simulink model "Model"  (R2024b)
settings: Solver=ode45  StartTime=0.0  StopTime=10  MaxStep=0.001  RelTol=1e-3
InitFcn:
  | Design
values from neighbouring files (symbols this model uses):
  Kw = 1 / Tw    (= 7.14285714286)    [Design.m]
  Mp = 0.3    [Design.m]
  P = (1 / (N * s)) * (kdrv * Kt * (Jb * s^2 + Bb * s + k))      / ((Req * D_tau_prime)      + Kt * Ke * (Jb * s^2 + Bb * s + k))    [Design.m]
  Ref = 50    [Design.m]
undefined symbols (not defined in the file or in its folder): daq, drv, ElecDyn, gbox, InternalTs, Kd, Ki, Kp, MechDyn, mld, mot, rads2rpm, sens, Tau_sf, Tl
libraries: simulink_extras x5
settings Model: Creator=Banaan  LastModifiedBy=Banaan

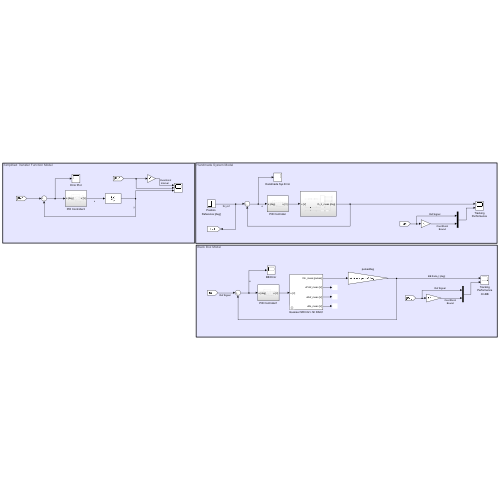
[thumbnail: Simulink's stored preview of the top-level diagram]
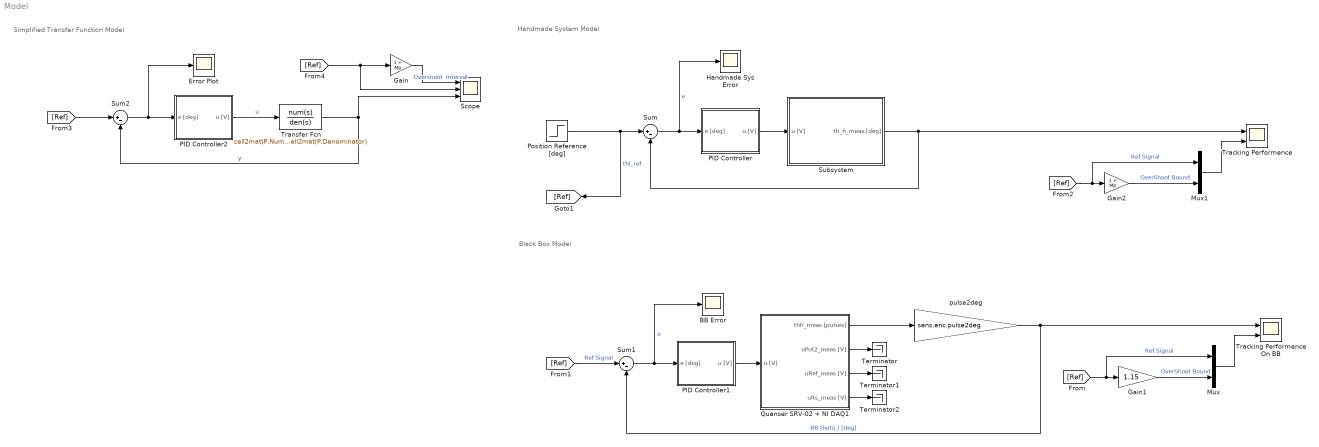
== system Model ==
  note: Simplified Transfer Function Model
  note: Handmade System Model
  note: Black Box Model
  BB Error : Scope
  Error Plot : Scope
  Gain : Gain  Gain=1 + Mp
  Gain1 : Gain  Gain=1.15
  Gain2 : Gain  Gain=1 + Mp
  Handmade Sys Error : Scope
  Mux : Mux  Inputs=2
  Mux1 : Mux  Inputs=2
  PID Controller : Subsystem
  PID Controller1 : Subsystem
  PID Controller2 : Subsystem
  Position Reference [deg] : Step  After=Ref  SampleTime=0
  Quanser SRV-02 + NI DAQ1 : Subsystem  mask(Quanser SRV-02 (with resonant load) + NI DAQ){Ts=0.001, fricType=Coulomb + viscous, lockShaft=off, beamInitPos=10}
      mask prompts: Ts "NI DAQ Sample Time:"; fricType "Friction model"; lockShaft "Lock motor shaft"; beamInitPos "Beam initial position [deg]:"
      mask help: Quanser SRV-02 (with resonant load) + NI DAQ model.
      mask init:
      | %%
      | % Riccardo Antonello (riccardo.antonello@unipd.it)
      | %
      | % April 28, 2020
      | %
      | % Dept. of Information Engineering, University of Padova
      | %
      | 
      | %%  Conversion gains
      | deg2rad = pi/180;                   %   [deg]   -> [rad]
      | rad2deg = 180/pi;                   %   [rad]   -> [deg]
      | 
      | 
      | %%  Sensors data
      | 
      | %   shunt resistor
      | sens.curr.Rs = 0.5;   
      | 
      | %   Hewlett-Packard HEDS-5540#A06 optical encoder
      | sens.enc.ppr = 500*4;                                                   %   pulses per rotation
      | sens.enc.pulse2deg = 360/sens.enc.ppr;                                  %   [pulses] -> [deg]
      | sens.enc.pulse2rad = 2*pi/sens.enc.ppr;                                 %   [pulses] -> [rad]
      | sens.enc.deg2pulse = sens.enc.ppr/360;                                  %   [deg] -> [pulses]
      | sens.enc.rad2pulse = sens.enc.ppr/2/pi;                                 %   [rad] -> [pulses]
      | 
      | %   potentiometer 2 (Spectrol 357-0-0-103) - installed on hub
      | sens.pot2.range.R      = 10e3;                                          %   ohmic value range 
      | sens.pot2.range.V      = 5;                                             %   voltage range
      | sens.pot2.range.th_deg = 340;                                           %   angle range [deg]
      | sens.pot2.range.th     = sens.pot2.range.th_deg * deg2rad;              %   angle range [rad]                           
      | sens.pot2.deg2V        = sens.pot2.range.V / sens.pot2.range.th_deg;    %   sensitivity [V/deg]
      | sens.pot2.rad2V        = sens.pot2.range.V / sens.pot2.range.th;        %   sensitivity [V/rad]
      | sens.pot2.V2deg        = 1/sens.pot2.deg2V;                             %   conversion gain [V] -> [deg]
      | sens.pot2.V2rad        = 1/sens.pot2.rad2V;                             %   conversion gain [V] -> [rad]
      | sens.pot2.noise.var    = 3.5e-7;                                        %   out noise variance [V^2]
      | 
      | 
      | %%  Data acquisition board (daq) data
      | 
      | %   NI PCI-6221 DAC data
      | daq.dac.bits = 16;                                  %   resolution (bits)
      | daq.dac.fs   = 10;                                  %   full scale 
      | daq.dac.q    = 2*daq.dac.fs/(2^daq.dac.bits-1);     %	quantization
      | 
      | %   NI PCI-6221 ADC data
      | daq.adc.bits = 16;                                  %   resolution (bits)
      | daq.adc.fs   = 10;                                  %   full scale (as set in SLDRT Analog Input block)
      | daq.adc.q    = 2*daq.adc.fs/(2^daq.adc.bits-1);     %   quantization   
      | 
      | 
      | %%  Set beam initial position
      | % SRV02Handle = find_system(gcb, ...
      | %     'LookUnderMasks', 'on', ...
      | %     'FindAll', 'on', ...
      | %     'FollowLinks', 'on', ...
      | %     'SearchDepth', '1', ...
      | %     'BlockType', 'ModelReference', ...
      | %     'Name', 'Quanser SRV-02');
      | %
      | % %get_param(SRV02Handle, 'InstanceParameters')
      | % InstanceParams = get_param(SRV02Handle, 'InstanceParameters');
      | % for k = 1:length(InstanceParams)
      | %     if strcmp(InstanceParams(k).Name, 'thb0')
      | %         if lockShaft
      | %             InstanceParams(k).Value = sprintf('%f', beamInitPos);
      | %         else
      | %             InstanceParams(k).Value = sprintf('%f', 0);    
      | %         end
      | %         set_param(SRV02Handle, 'InstanceParameters', InstanceParams);
      | %         break;
      | %     end
      | % end
      | 
      | if lockShaft
      |     thb0 = beamInitPos;
      | else
      |     thb0 = 0;    
      | end
      | 
      | 
      | %%  Mask initialization
      | if lockShaft
      |     
      |     %   find Inport handle
      |     InPortHandle = find_system(gcb, ...
      |         'LookUnderMasks', 'on', ...
      |         'FindAll', 'on', ...
      |         'FollowLinks', 'on', ...
      |         'SearchDepth', '1', ...
      |         'BlockType', 'Inport', ...
      |         'Name', 'u [V]');
      |     
      |     if ~isempty(InPortHandle)
      |     
      |         %   find DAC handle
      |         DACHandle = find_system(gcb, ...
      |             'LookUnderMasks', 'on', ...
      |             'FindAll', 'on', ...
      |             'FollowLinks', 'on', ...
      |             'SearchDepth', '1', ...
      |             'BlockType', 'SubSystem', ...
      |             'Name', 'DAC');  
      | 
      |         %   remove Inport output connection   
      |         InportConn = get_param(InPortHandle, 'PortConnectivity');
      |         delete_line(gcb, InportConn.Position);
      | 
      |         %   remove Inport block
      |         delete_block(InPortHandle);
      | 
      |         %   add Constant block
      |         ConstantHandle = add_block( ...
      |             'simulink/Sources/Constant', [gcb, '/u [V]'], ...
      |             'Position', [20   -37    50   -23], ...
      |             'Value', '0');
      | 
      |         %   connect Constant to DAC block
      |         DACPortHandles = get_param(DACHandle, 'PortHandles');
      |         ConstantPortHandles = get_param(ConstantHandle, 'PortHandles');
      |         add_line(gcb, ConstantPortHandles.Outport(1), DACPortHandles.Inport(1));
      |     
      |     end
      |     
      | else
      |     
      |     %   find Constant handle
      |     ConstantHandle = find_system(gcb, ...
      |         'LookUnderMasks', 'on', ...
      |         'FindAll', 'on', ...
      |         'FollowLinks', 'on', ...
      |         'SearchDepth', '1', ...
      |         'BlockType', 'Constant', ...
      |         'Name', 'u [V]');
      |     
      |     if ~isempty(ConstantHandle)
      |     
      |         %   find DAC handle
      |         DACHandle = find_system(gcb, ...
      |             'LookUnderMasks', 'on', ...
      |             'FindAll', 'on', ...
      |             'FollowLinks', 'on', ...
      |             'SearchDepth', '1', ...
      |             'BlockType', 'SubSystem', ...
      |             'Name', 'DAC');  
      |  
      |         %   remove Constant output connection   
      |         ConstantConn = get_param(ConstantHandle, 'PortConnectivity');
      |         delete_line(gcb, ConstantConn.Position);
      | 
      |         %   remove Inport block
      |         delete_block(ConstantHandle);   
      | 
      |         %   add Inport block
      |         InportHandle = add_block( ...
      |             'simulink/Sources/In1', [gcb, '/u [V]'], ...
      |             'Position', [20   -37    50   -23], ...
      |             'Port', '1');
      | 
      |         %   connect Constant to DAC block
      |         DACPortHandles = get_param(DACHandle, 'PortHandles');
      |         InportPortHandles = get_param(InportHandle, 'PortHandles');
      |         add_line(gcb, InportPortHandles.Outport(1), DACPortHandles.Inport(1));
      |     
      |      end
      |     
      | end
      mask Help:
      | Riccardo Antonello (antonello@dei.unipd.it)
      | 
      | April 28, 2020
      | 
      | Dept. of Information Engineering, University of Padova
      mask TypeOptions fricType: Coulomb + viscous | Karnopp
      mask Callback lockShaft:
      | %   get status of check box
      | lockShaft = get_param(gcb, 'lockShaft');
      | 
      | %   get current value of MaskVisibilities property
      | maskVisibilities = get_param(gcb, 'MaskVisibilities');
      | 
      | %   set visibility of the dialog box element
      | if strcmp(lockShaft, 'on')
      |     maskVisibilities{4} = 'on';
      | else
      |     maskVisibilities{4} = 'off';
      | end
      | 
      | % Set the 'MaskVisibilities' property for each parameter in mask
      | set_param( gcb, 'MaskVisibilities', maskVisibilities);
  Scope : Scope  NumInputPorts=3
  Subsystem : Subsystem
  Sum : Sum  Inputs=|+-
  Sum1 : Sum  Inputs=|+-
  Sum2 : Sum  Inputs=|+-
  Terminator : Terminator
  Terminator1 : Terminator
  Terminator2 : Terminator
  Tracking Performence : Scope  NumInputPorts=2
  Tracking Performence On BB : Scope  NumInputPorts=2
  Transfer Fcn : TransferFcn  Numerator=cell2mat(P.Numerator)  Denominator=cell2mat(P.Denominator)
  pulse2deg : Gain  Gain=sens.enc.pulse2deg
  wires:
  PID Controller/1(u [V]) -> Subsystem/1(u [V])
  Sum/1 -> PID Controller/1(e [deg]), Handmade Sys Error/1  "e"
  Subsystem/1(th_h_meas [deg]) -> Tracking Performence/1, Sum/2
  Position Reference [deg]/1 -> [Ref], Sum/1  "thl_ref"
  Quanser SRV-02 + NI DAQ1/1(thh_meas [pulses]) -> pulse2deg/1
  pulse2deg/1 -> Tracking Performence On BB/1, Sum1/2  "BB theta_l [deg]"
  Sum1/1 -> PID Controller1/1(e [deg]), BB Error/1  "e"
  PID Controller1/1(u [V]) -> Quanser SRV-02 + NI DAQ1/1(u [V])
  Gain1/1 -> Mux/2  "OverShoot Bound"
  [Ref] -> Mux/1, Gain1/1  "Ref Signal"
  Mux/1 -> Tracking Performence On BB/2
  [Ref] -> Sum1/1  "Ref Signal"
  Mux1/1 -> Tracking Performence/2
  [Ref] -> Gain2/1, Mux1/1  "Ref Signal"
  Gain2/1 -> Mux1/2  "OverShoot Bound"
  PID Controller2/1(u [V]) -> Transfer Fcn/1  "u"
  [Ref] -> Sum2/1
  Sum2/1 -> Error Plot/1, PID Controller2/1(e [deg])
  Transfer Fcn/1 -> Sum2/2, Scope/3  "y"
  Gain/1 -> Scope/1  "Overshoot  Interval"
  [Ref] -> Scope/2, Gain/1
  Quanser SRV-02 + NI DAQ1/3(uRef_meas [V]) -> Terminator1/1
  Quanser SRV-02 + NI DAQ1/2(uPot2_meas [V]) -> Terminator/1
  Quanser SRV-02 + NI DAQ1/4(uRs_meas [V]) -> Terminator2/1

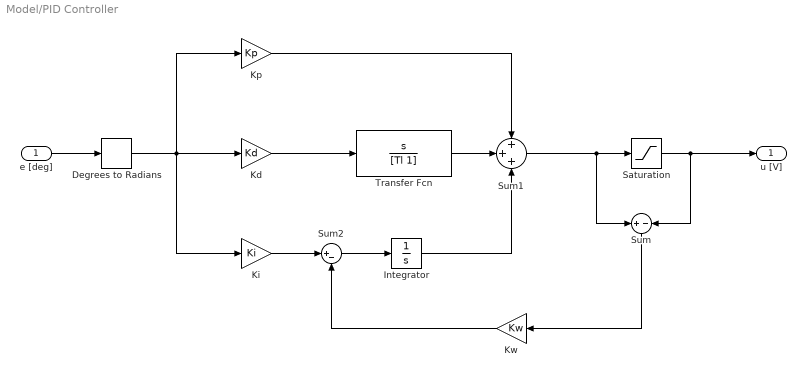
== system Model/PID Controller ==
  e [deg] : Inport
  Degrees to Radians : simulink_extras/Transformations/Degrees to Radians
  Integrator : Integrator
  Kd : Gain  Gain=Kd
  Ki : Gain  Gain=Ki
  Kp : Gain  Gain=Kp
  Kw : Gain  Gain=Kw
  Saturation : Saturate  UpperLimit=daq.dac.fs  LowerLimit=-daq.dac.fs
  Sum : Sum  Inputs=+|-
  Sum1 : Sum  Inputs=+++
  Sum2 : Sum  Inputs=|+-
  Transfer Fcn : TransferFcn  Numerator=[1 0]  Denominator=[Tl 1]
  u [V] : Outport
  wires:
  Integrator/1 -> Sum1/3
  Sum2/1 -> Integrator/1
  Sum1/1 -> Sum/1, Saturation/1
  Ki/1 -> Sum2/1
  Kw/1 -> Sum2/2
  Kp/1 -> Sum1/1
  Sum/1 -> Kw/1
  Transfer Fcn/1 -> Sum1/2
  e [deg]/1 -> Degrees to Radians/1
  Kd/1 -> Transfer Fcn/1
  Saturation/1 -> u [V]/1, Sum/2
  Degrees to Radians/1 -> Kp/1, Kd/1, Ki/1

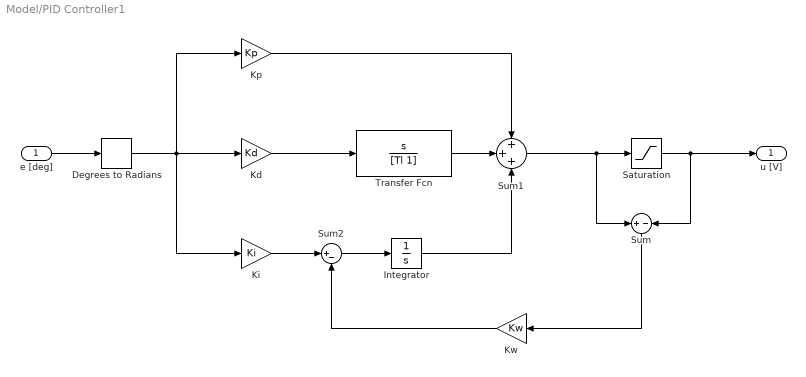
== system Model/PID Controller1 ==
  e [deg] : Inport
  Degrees to Radians : simulink_extras/Transformations/Degrees to Radians
  Integrator : Integrator
  Kd : Gain  Gain=Kd
  Ki : Gain  Gain=Ki
  Kp : Gain  Gain=Kp
  Kw : Gain  Gain=Kw
  Saturation : Saturate  UpperLimit=daq.dac.fs  LowerLimit=-daq.dac.fs
  Sum : Sum  Inputs=+|-
  Sum1 : Sum  Inputs=+++
  Sum2 : Sum  Inputs=|+-
  Transfer Fcn : TransferFcn  Numerator=[1 0]  Denominator=[Tl 1]
  u [V] : Outport
  wires:
  Kp/1 -> Sum1/1
  Degrees to Radians/1 -> Kp/1, Kd/1, Ki/1
  e [deg]/1 -> Degrees to Radians/1
  Saturation/1 -> u [V]/1, Sum/2
  Transfer Fcn/1 -> Sum1/2
  Sum2/1 -> Integrator/1
  Kd/1 -> Transfer Fcn/1
  Sum1/1 -> Sum/1, Saturation/1
  Sum/1 -> Kw/1
  Integrator/1 -> Sum1/3
  Kw/1 -> Sum2/2
  Ki/1 -> Sum2/1

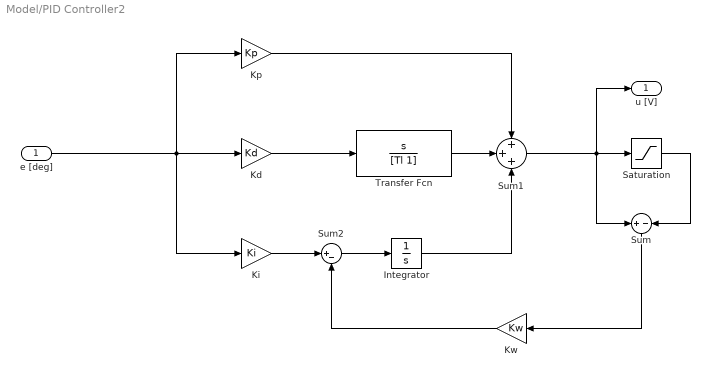
== system Model/PID Controller2 ==
  e [deg] : Inport
  Integrator : Integrator
  Kd : Gain  Gain=Kd
  Ki : Gain  Gain=Ki
  Kp : Gain  Gain=Kp
  Kw : Gain  Gain=Kw
  Saturation : Saturate  UpperLimit=daq.dac.fs  LowerLimit=-daq.dac.fs
  Sum : Sum  Inputs=+|-
  Sum1 : Sum  Inputs=+++
  Sum2 : Sum  Inputs=|+-
  Transfer Fcn : TransferFcn  Numerator=[1 0]  Denominator=[Tl 1]
  u [V] : Outport
  wires:
  Sum1/1 -> u [V]/1, Sum/1, Saturation/1
  Kp/1 -> Sum1/1
  Kd/1 -> Transfer Fcn/1
  Ki/1 -> Sum2/1
  e [deg]/1 -> Kp/1, Kd/1, Ki/1
  Saturation/1 -> Sum/2
  Sum2/1 -> Integrator/1
  Sum/1 -> Kw/1
  Kw/1 -> Sum2/2
  Transfer Fcn/1 -> Sum1/2
  Integrator/1 -> Sum1/3

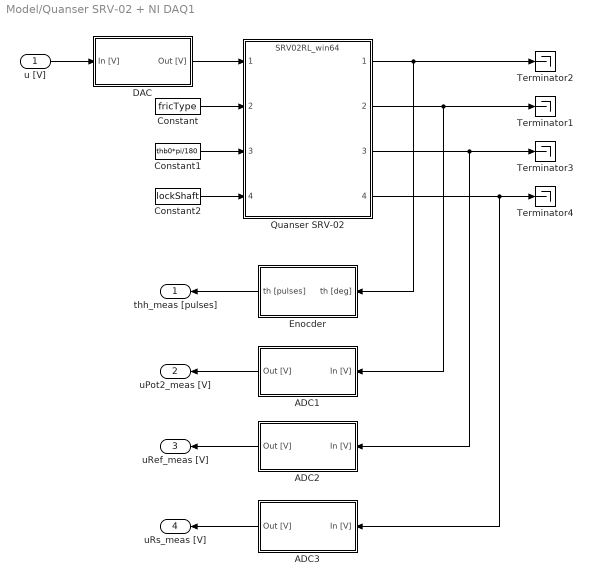
== system Model/Quanser SRV-02 + NI DAQ1 ==
  u [V] : Inport
  ADC1 : Subsystem
  ADC2 : Subsystem
  ADC3 : Subsystem
  Constant : Constant  Value=fricType
  Constant1 : Constant  Value=thb0*pi/180  SampleTime=Inf
  Constant2 : Constant  Value=lockShaft  SampleTime=Inf
  DAC : Subsystem
  Enocder : Subsystem
  Quanser SRV-02 : ModelReference  ModelNameDialog=SRV02RL_win64.slxp  ModelReferenceVersion=1.76  CopyOfModelProtected=on
  Terminator{1..4} (4 alike) : Terminator
  thh_meas [pulses] : Outport
  uPot2_meas [V] : Outport  Port=2
  uRef_meas [V] : Outport  Port=3
  uRs_meas [V] : Outport  Port=4
  wires:
  Enocder/1(th [pulses]) -> thh_meas [pulses]/1
  ADC3/1(Out [V]) -> uRs_meas [V]/1
  DAC/1(Out [V]) -> Quanser SRV-02/1
  Quanser SRV-02/2 -> ADC1/1(In [V]), Terminator1/1
  Quanser SRV-02/1 -> Terminator2/1, Enocder/1(th [deg])
  Constant/1 -> Quanser SRV-02/2
  Quanser SRV-02/3 -> ADC2/1(In [V]), Terminator3/1
  ADC1/1(Out [V]) -> uPot2_meas [V]/1
  Constant1/1 -> Quanser SRV-02/3
  Constant2/1 -> Quanser SRV-02/4
  Quanser SRV-02/4 -> ADC3/1(In [V]), Terminator4/1
  ADC2/1(Out [V]) -> uRef_meas [V]/1
  u [V]/1 -> DAC/1(In [V])

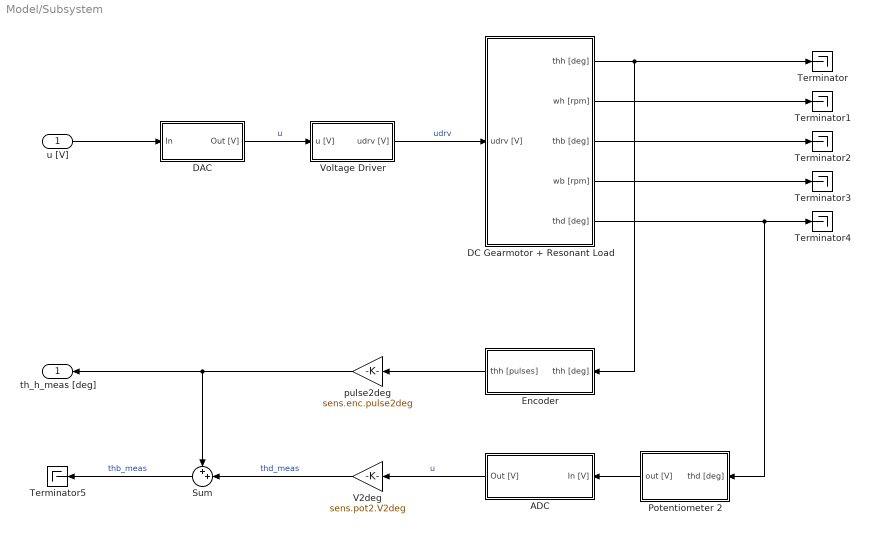
== system Model/Subsystem ==
  u [V] : Inport
  ADC : Subsystem
  DAC : Subsystem
  DC Gearmotor + Resonant Load : Subsystem
  Encoder : Subsystem
  Potentiometer 2 : Subsystem
  Sum : Sum  Inputs=++|
  Terminator{,1..5} (6 alike) : Terminator
  V2deg : Gain  Gain=sens.pot2.V2deg
  Voltage Driver : Subsystem
  pulse2deg : Gain  Gain=sens.enc.pulse2deg
  th_h_meas [deg] : Outport
  wires:
  DAC/1(Out [V]) -> Voltage Driver/1(u [V])  "u"
  Encoder/1(thh [pulses]) -> pulse2deg/1
  u [V]/1 -> DAC/1(In)
  Voltage Driver/1(udrv [V]) -> DC Gearmotor + Resonant Load/1(udrv [V])  "udrv"
  pulse2deg/1 -> th_h_meas [deg]/1, Sum/1
  DC Gearmotor + Resonant Load/1(thh [deg]) -> Terminator/1, Encoder/1(thh [deg])
  ADC/1(Out [V]) -> V2deg/1  "u"
  V2deg/1 -> Sum/2  "thd_meas"
  Sum/1 -> Terminator5/1  "thb_meas"
  DC Gearmotor + Resonant Load/5(thd [deg]) -> Potentiometer 2/1(thd [deg]), Terminator4/1
  DC Gearmotor + Resonant Load/2(wh [rpm]) -> Terminator1/1
  DC Gearmotor + Resonant Load/3(thb [deg]) -> Terminator2/1
  DC Gearmotor + Resonant Load/4(wb [rpm]) -> Terminator3/1
  Potentiometer 2/1(out [V]) -> ADC/1(In [V])

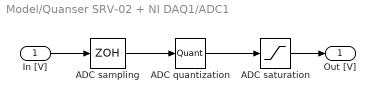
== system Model/Quanser SRV-02 + NI DAQ1/ADC1 ==
  In [V] : Inport
  ADC quantization : Quantizer  QuantizationInterval=daq.adc.q
  ADC sampling : ZeroOrderHold  SampleTime=Ts
  ADC saturation : Saturate  UpperLimit=daq.adc.fs  LowerLimit=-daq.adc.fs
  Out [V] : Outport
  wires:
  ADC saturation/1 -> Out [V]/1
  ADC sampling/1 -> ADC quantization/1
  In [V]/1 -> ADC sampling/1
  ADC quantization/1 -> ADC saturation/1

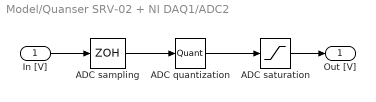
== system Model/Quanser SRV-02 + NI DAQ1/ADC2 ==
  In [V] : Inport
  ADC quantization : Quantizer  QuantizationInterval=daq.adc.q
  ADC sampling : ZeroOrderHold  SampleTime=Ts
  ADC saturation : Saturate  UpperLimit=daq.adc.fs  LowerLimit=-daq.adc.fs
  Out [V] : Outport
  wires:
  ADC quantization/1 -> ADC saturation/1
  In [V]/1 -> ADC sampling/1
  ADC sampling/1 -> ADC quantization/1
  ADC saturation/1 -> Out [V]/1

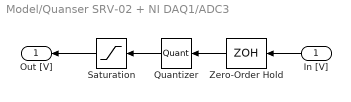
== system Model/Quanser SRV-02 + NI DAQ1/ADC3 ==
  In [V] : Inport
  Quantizer : Quantizer  QuantizationInterval=daq.adc.q
  Saturation : Saturate  UpperLimit=daq.adc.fs  LowerLimit=-daq.adc.fs
  Zero-Order Hold : ZeroOrderHold  SampleTime=Ts
  Out [V] : Outport
  wires:
  Saturation/1 -> Out [V]/1
  In [V]/1 -> Zero-Order Hold/1
  Quantizer/1 -> Saturation/1
  Zero-Order Hold/1 -> Quantizer/1

== system Model/Quanser SRV-02 + NI DAQ1/DAC ==
  In [V] : Inport
  Quantizer : Quantizer  QuantizationInterval=daq.dac.q
  Saturation : Saturate  UpperLimit=daq.dac.fs  LowerLimit=-daq.dac.fs
  Zero-Order Hold : ZeroOrderHold  SampleTime=Ts
  Out [V] : Outport
  wires:
  Quantizer/1 -> Saturation/1
  In [V]/1 -> Zero-Order Hold/1
  Zero-Order Hold/1 -> Quantizer/1
  Saturation/1 -> Out [V]/1

== system Model/Quanser SRV-02 + NI DAQ1/Enocder ==
  th [deg] : Inport
  Quantizer : Quantizer  QuantizationInterval=sens.enc.pulse2deg
  Zero-Order Hold : ZeroOrderHold  SampleTime=Ts
  deg2pulse : Gain  Gain=sens.enc.deg2pulse
  th [pulses] : Outport
  wires:
  Quantizer/1 -> deg2pulse/1
  th [deg]/1 -> Zero-Order Hold/1
  Zero-Order Hold/1 -> Quantizer/1
  deg2pulse/1 -> th [pulses]/1

== system Model/Subsystem/ADC ==
  In [V] : Inport
  ADC Quantization : Quantizer  QuantizationInterval=daq.adc.q
  ADC Sampling : ZeroOrderHold  SampleTime=InternalTs
  ADC Saturation : Saturate  UpperLimit=daq.adc.fs  LowerLimit=-daq.adc.fs
  Out [V] : Outport
  wires:
  In [V]/1 -> ADC Sampling/1
  ADC Saturation/1 -> Out [V]/1
  ADC Sampling/1 -> ADC Quantization/1
  ADC Quantization/1 -> ADC Saturation/1

== system Model/Subsystem/DAC ==
  In : Inport
  DAC Quantization : Quantizer  QuantizationInterval=daq.dac.q
  DAC Saturation : Saturate  UpperLimit=daq.dac.fs  LowerLimit=-daq.dac.fs
  DAC ZOH : ZeroOrderHold  SampleTime=InternalTs
  Out [V] : Outport
  wires:
  DAC Quantization/1 -> DAC Saturation/1
  DAC ZOH/1 -> DAC Quantization/1
  DAC Saturation/1 -> Out [V]/1
  In/1 -> DAC ZOH/1

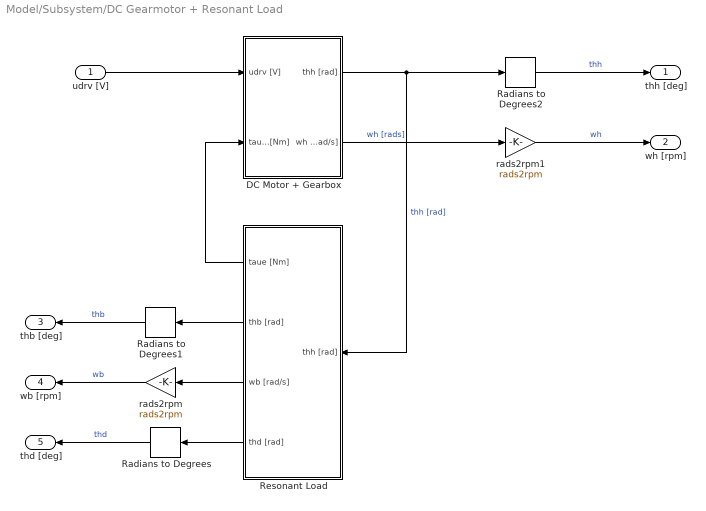
== system Model/Subsystem/DC Gearmotor + Resonant Load ==
  udrv [V] : Inport
  DC Motor + Gearbox : Subsystem
  Radians to Degrees : simulink_extras/Transformations/Radians to Degrees
  Radians to Degrees1 : simulink_extras/Transformations/Radians to Degrees
  Radians to Degrees2 : simulink_extras/Transformations/Radians to Degrees
  Resonant Load : Subsystem
  rads2rpm : Gain  Gain=rads2rpm
  rads2rpm1 : Gain  Gain=rads2rpm
  thh [deg] : Outport
  wh [rpm] : Outport  Port=2
  thb [deg] : Outport  Port=3
  wb [rpm] : Outport  Port=4
  thd [deg] : Outport  Port=5
  wires:
  Radians to Degrees/1 -> thd [deg]/1  "thd"
  Resonant Load/4(thd [rad]) -> Radians to Degrees/1
  DC Motor + Gearbox/2(wh [rad/s]) -> rads2rpm1/1  "wh [rads]"
  Resonant Load/2(thb [rad]) -> Radians to Degrees1/1
  Resonant Load/1(taue [Nm]) -> DC Motor + Gearbox/2(taue [Nm])
  DC Motor + Gearbox/1(thh [rad]) -> Resonant Load/1(thh [rad]), Radians to Degrees2/1  "thh [rad]"
  Resonant Load/3(wb [rad/s]) -> rads2rpm/1
  Radians to Degrees2/1 -> thh [deg]/1  "thh"
  rads2rpm/1 -> wb [rpm]/1  "wb"
  Radians to Degrees1/1 -> thb [deg]/1  "thb"
  udrv [V]/1 -> DC Motor + Gearbox/1(udrv [V])
  rads2rpm1/1 -> wh [rpm]/1  "wh"

== system Model/Subsystem/Encoder ==
  thh [deg] : Inport
  Encoder Quantization : Quantizer  QuantizationInterval=daq.adc.q
  Encoder Sampling : ZeroOrderHold  SampleTime=InternalTs
  deg2pulse : Gain  Gain=sens.enc.deg2pulse
  thh [pulses] : Outport
  wires:
  Encoder Sampling/1 -> Encoder Quantization/1
  Encoder Quantization/1 -> deg2pulse/1
  thh [deg]/1 -> Encoder Sampling/1
  deg2pulse/1 -> thh [pulses]/1

== system Model/Subsystem/Potentiometer 2 ==
  thd [deg] : Inport
  Sensor Output Noise [V] : RandomNumber  Variance=sens.pot2.noise.var  SampleTime=InternalTs
  Sum1 : Sum  Inputs=++|
  deg2V : Gain  Gain=sens.pot2.deg2V
  out [V] : Outport
  wires:
  deg2V/1 -> Sum1/2
  Sum1/1 -> out [V]/1  "thb_meas"
  thd [deg]/1 -> deg2V/1
  Sensor Output Noise [V]/1 -> Sum1/1

== system Model/Subsystem/Voltage Driver ==
  u [V] : Inport
  Driver Dynamics : TransferFcn  Numerator=drv.dcgain  Denominator=[drv.Tc, 1]
  Driver Saturation : Saturate  UpperLimit=drv.outmax  LowerLimit=-drv.outmax
  udrv [V] : Outport
  wires:
  Driver Dynamics/1 -> Driver Saturation/1
  u [V]/1 -> Driver Dynamics/1
  Driver Saturation/1 -> udrv [V]/1

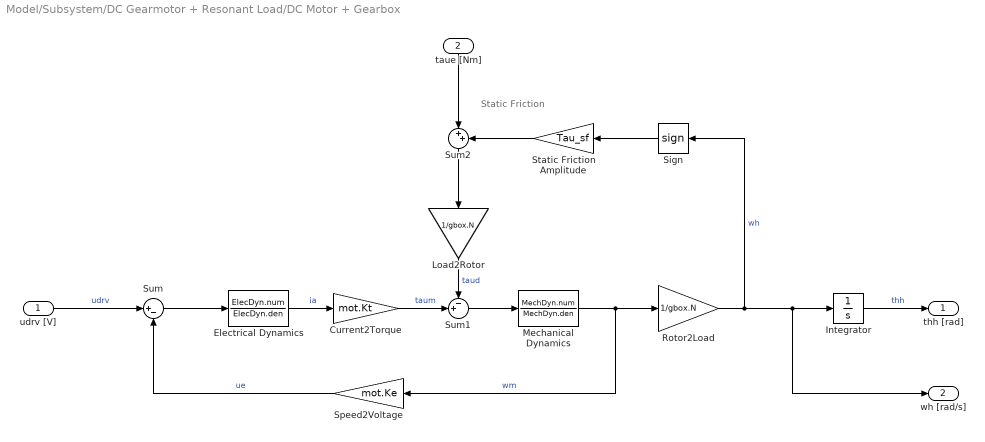
== system Model/Subsystem/DC Gearmotor + Resonant Load/DC Motor + Gearbox ==
  note: Static Friction
  udrv [V] : Inport
  taue [Nm] : Inport  Port=2
  Current2Torque : Gain  Gain=mot.Kt
  Electrical Dynamics : TransferFcn  Numerator=ElecDyn.num  Denominator=ElecDyn.den
  Integrator : Integrator
  Load2Rotor : Gain  Gain=1/gbox.N
  Mechanical Dynamics : TransferFcn  Numerator=MechDyn.num  Denominator=MechDyn.den
  Rotor2Load : Gain  Gain=1/gbox.N
  Sign : Signum  ZeroCross=off
  Speed2Voltage : Gain  Gain=mot.Ke
  Static Friction Amplitude : Gain  Gain=Tau_sf
  Sum : Sum  Inputs=|+-
  Sum1 : Sum  Inputs=-+|
  Sum2 : Sum  Inputs=|++
  thh [rad] : Outport
  wh [rad/s] : Outport  Port=2
  wires:
  Rotor2Load/1 -> wh [rad/s]/1, Integrator/1, Sign/1  "wh"
  Electrical Dynamics/1 -> Current2Torque/1  "ia"
  Sum1/1 -> Mechanical Dynamics/1
  Speed2Voltage/1 -> Sum/2  "ue"
  Load2Rotor/1 -> Sum1/1  "taud"
  Mechanical Dynamics/1 -> Speed2Voltage/1, Rotor2Load/1  "wm"
  Sum/1 -> Electrical Dynamics/1
  Integrator/1 -> thh [rad]/1  "thh"
  Current2Torque/1 -> Sum1/2  "taum"
  Sign/1 -> Static Friction Amplitude/1
  Static Friction Amplitude/1 -> Sum2/2
  udrv [V]/1 -> Sum/1  "udrv"
  Sum2/1 -> Load2Rotor/1
  taue [Nm]/1 -> Sum2/1

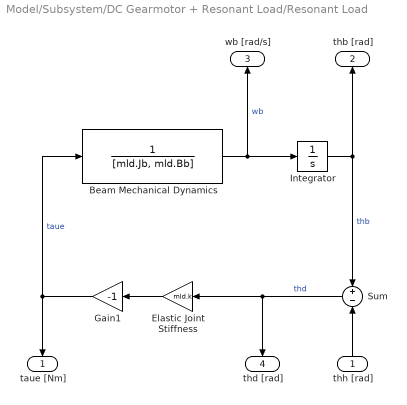
== system Model/Subsystem/DC Gearmotor + Resonant Load/Resonant Load ==
  thh [rad] : Inport
  Beam Mechanical Dynamics : TransferFcn  Denominator=[mld.Jb, mld.Bb]
  Elastic Joint Stiffness : Gain  Gain=mld.k
  Gain1 : Gain  Gain=-1
  Integrator : Integrator
  Sum : Sum  Inputs=+|-
  taue [Nm] : Outport
  thb [rad] : Outport  Port=2
  wb [rad/s] : Outport  Port=3
  thd [rad] : Outport  Port=4
  wires:
  Integrator/1 -> thb [rad]/1, Sum/1  "thb"
  Beam Mechanical Dynamics/1 -> wb [rad/s]/1, Integrator/1  "wb"
  Gain1/1 -> Beam Mechanical Dynamics/1, taue [Nm]/1  "taue"
  Elastic Joint Stiffness/1 -> Gain1/1
  Sum/1 -> Elastic Joint Stiffness/1, thd [rad]/1  "thd"
  thh [rad]/1 -> Sum/2
